simulink model "Exercise_P85"  (R2023b)
settings: Solver=VariableStepAuto  StartTime=0.0  StopTime=10.0  RelTol=1e-3
values from neighbouring files (symbols this model uses):
  K1 = 0.1    [Ex_P85.m]
  K2 = 0.533    [Ex_P85.m]
  K3 = 1    [Ex_P85.m]
settings Model: Creator=mdhel  LastModifiedBy=mdhel

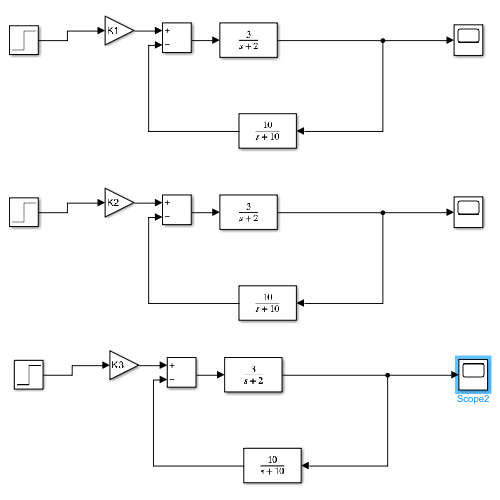
[thumbnail: Simulink's stored preview of the top-level diagram]
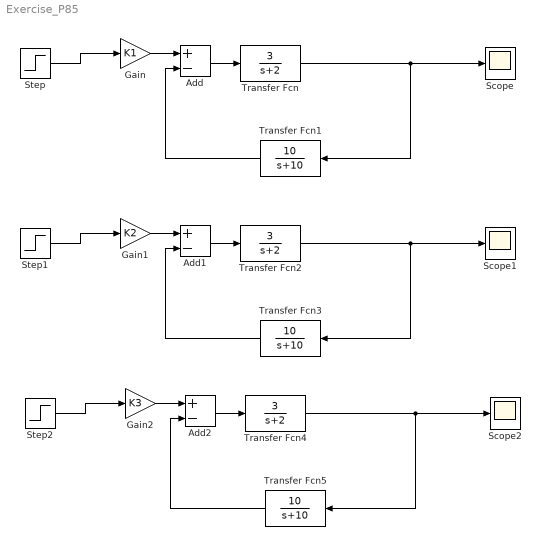
== system Exercise_P85 ==
  Add : Sum  Inputs=+-
  Add1 : Sum  Inputs=+-
  Add2 : Sum  Inputs=+-
  Gain : Gain  Gain=K1
  Gain1 : Gain  Gain=K2
  Gain2 : Gain  Gain=K3
  Scope : Scope
  Scope1 : Scope
  Scope2 : Scope
  Step : Step  SampleTime=0
  Step1 : Step  SampleTime=0
  Step2 : Step  SampleTime=0
  Transfer Fcn : TransferFcn  Numerator=[3]  Denominator=[1 2]
  Transfer Fcn1 : TransferFcn  Numerator=[10]  Denominator=[1 10]
  Transfer Fcn2 : TransferFcn  Numerator=[3]  Denominator=[1 2]
  Transfer Fcn3 : TransferFcn  Numerator=[10]  Denominator=[1 10]
  Transfer Fcn4 : TransferFcn  Numerator=[3]  Denominator=[1 2]
  Transfer Fcn5 : TransferFcn  Numerator=[10]  Denominator=[1 10]
  wires:
  Gain/1 -> Add/1
  Step/1 -> Gain/1
  Transfer Fcn/1 -> Transfer Fcn1/1, Scope/1
  Add/1 -> Transfer Fcn/1
  Transfer Fcn1/1 -> Add/2
  Gain1/1 -> Add1/1
  Step1/1 -> Gain1/1
  Transfer Fcn2/1 -> Transfer Fcn3/1, Scope1/1
  Add1/1 -> Transfer Fcn2/1
  Transfer Fcn3/1 -> Add1/2
  Gain2/1 -> Add2/1
  Step2/1 -> Gain2/1
  Transfer Fcn4/1 -> Transfer Fcn5/1, Scope2/1
  Add2/1 -> Transfer Fcn4/1
  Transfer Fcn5/1 -> Add2/2
